simulink model "ACC_bicycleModel"  (R2022a)
settings: Solver=FixedStepAuto  StartTime=0.0  StopTime=T  RelTol=1e-3
values from neighbouring files (symbols this model uses):
  o0_ego_1 = 0    [PreRun.m]
  o0_lead = 0    [PreRun.m]
  t_gap = 1.4    [PreRun.m]
  Ts = 1e-2    (= 0.01)    [PreRun.m]
  v0_ego_1 = 20/9    (= 2.22222222222)    [PreRun.m]
  v0_lead = 25/9    (= 2.77777777778)    [PreRun.m]
  v_set = 30    [PreRun.m]
  x0_ego_1 = x0_lead - (10 + t_gap*v0_ego_1)    (= 56.8888888889)    [PreRun.m]
  x0_ego_2 = x0_ego_1 - (10 + t_gap*v0_ego_2)    (= 43.7777777778)    [PreRun.m]
  x0_lead = 70    [PreRun.m]
  y0_ego_1 = 0    [PreRun.m]
  y0_lead = 0    [PreRun.m]
libraries: robotmobilelib x3, mpcadaslib x2
settings Model: Creator=The MathWorks, Inc.  LastModifiedBy=SAMEER TALWAR
settings SolverCC: AlgebraicLoopSolver=TrustRegion
settings DataIOCC: ReturnWorkspaceOutputs=off
settings DebuggingCC: UnconnectedInputMsg=warning  UnconnectedOutputMsg=warning  UnconnectedLineMsg=warning  SFMachineParentedDataDiag=warning  ArithmeticOperatorsInVariantConditions=warning
settings SFSimCC: SimUseLocalCustomCode=off  CustomCodeUndefinedFunction=UseInterfaceOnly
settings RTWCC: RTWUseLocalCustomCode=off
settings CodeAppCC: StateflowObjectComments=on

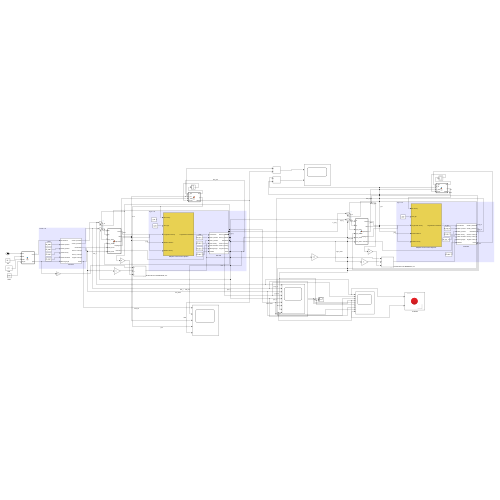
[thumbnail: Simulink's stored preview of the top-level diagram]
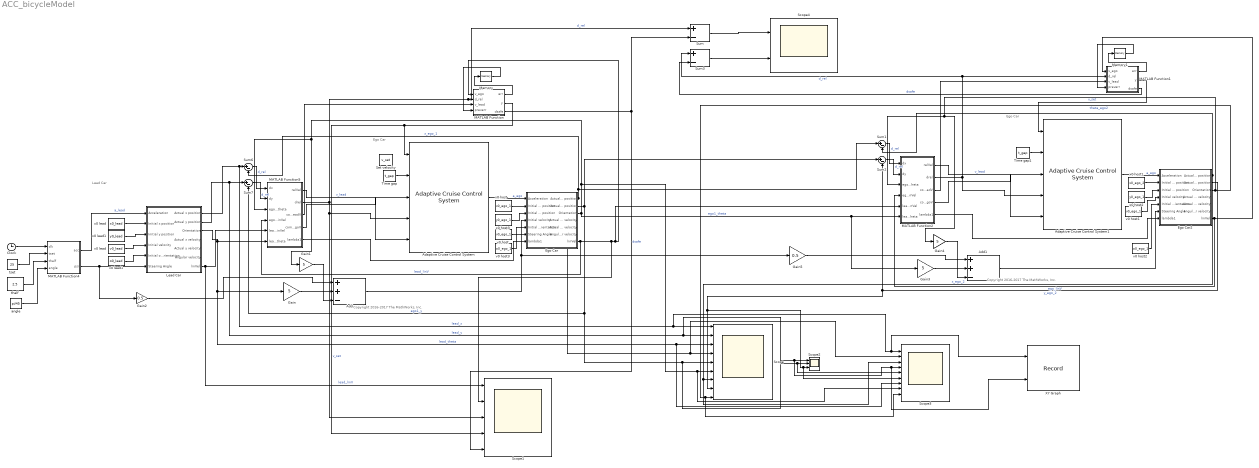
== system ACC_bicycleModel ==
  note: Lead Car
  note: Ego Car
  note: Copyright 2016-2017 The MathWorks, Inc.
  note: Ego Car
  note: Copyright 2016-2017 The MathWorks, Inc.
  Adaptive Cruise Control System : mpcadaslib/Adaptive Cruise Control System  EgoModel=tf(1,[0.5,1,0])  InitialEgoVelocity=20  DefaultSpacing=10  MaxVelocity=100  MinAcceleration=-30  amin_ext=off  MaxAcceleration=20  amax_ext=off  Ts=Ts  PredictionHorizon=30  ControllerBehavior=1.0  suboptimal=off  maxiter=10  datatypeopt=double  optmode=off  trackmode=off
  Adaptive Cruise Control System1 : mpcadaslib/Adaptive Cruise Control System  EgoModel=tf(1,[0.5,1,0])  InitialEgoVelocity=20  DefaultSpacing=10  MaxVelocity=100  MinAcceleration=-30  amin_ext=off  MaxAcceleration=20  amax_ext=off  Ts=Ts  PredictionHorizon=30  ControllerBehavior=1.0  suboptimal=off  maxiter=10  datatypeopt=double  optmode=off  trackmode=off
  Add : Sum  Inputs=++-
  Add1 : Sum  Inputs=++-
  Clock : Clock
  Ego Car : Subsystem
  Ego Car2 : Subsystem
  Gain{,1,3..4} (4 alike) : Gain  Gain=5
  Gain2 : Gain  Gain=0.5
  Gain5 : Gain  Gain=0.5
  Lead Car : Subsystem
  MATLAB Function : MATLAB Function  TreatAsAtomicUnit=on
  MATLAB Function1 : MATLAB Function  TreatAsAtomicUnit=on
  MATLAB Function2 : MATLAB Function  TreatAsAtomicUnit=on
  MATLAB Function4 : MATLAB Function  TreatAsAtomicUnit=on
  MATLAB Function5 : MATLAB Function  TreatAsAtomicUnit=on
  Memory : Memory
  Memory1 : Memory
  Scope : Scope  NumInputPorts=9
  Scope1 : Scope  NumInputPorts=5
  Scope2 : Scope  NumInputPorts=3
  Scope3 : Scope  NumInputPorts=9
  Scope4 : Scope  NumInputPorts=2
  Set velocity : Constant  Value=v_set  SampleTime=Ts
  Sum : Sum  Inputs=+-
  Sum{1..2,6..7} (4 alike) : Sum  Inputs=|+-
  Sum3 : Sum  Inputs=+-
  Time gap : Constant  Value=t_gap  SampleTime=Ts
  Time gap1 : Constant  Value=t_gap  SampleTime=Ts
  XY Graph : Record  FileSettingsInternal="{\"entries\":[{\"content\":{\"excelSettings\":{\"content\":{},\"type\":\"Streamout.ExcelSettings\"}},\"type\":\"Streamout.FileSettingStorage\",\"uuid\":\"e1ca2645-03e2-4b36-ae2b-66a36fe1bab2\"}],\"packageUris\":[\"http://schema.mathworks.com/mf0/streamout_blocks/R2020a\"],\"version\":\"1.0\"}"  Layout=[1 1]  SignalsInternal="{\"entries\":[{\"content\":{\"signals\":[{\"content\":{\"blockPath\":[\"ACC_bicycleModel/XY Graph\"],\"channel\":[],\"dimensions\":[1],\"domain\":\"ACC_bicycleModel/XY Graph\",\"lineColor\":\"#a2142f\",\"plots\":[1],\"port\":1,\"sid\":[],\"signalID\":18,\"signalName\":\"lead_x\"},\"type\":\"RecordBlkView.Signal\",\"uuid\":\"ab4e1985-af17-4664-8952-9c7faca9cf0c\"},{\"content\":{\"blockPath\":[\"ACC_bicycleModel/XY Graph\"],\"channel\":[],\"dimensions\":[1],\"domain\":\"ACC_bicycleModel/XY Graph\",\"lineColor\":\"#139fff\",\"plots\":[1],\"port\":2,\"sid\":[],\"signalID\":21,\"signalName\":\"lead_y\"},\"type\":\"RecordBlkView.Signal\",\"uuid\":\"8268d064-4b91-4bd3-a13e-a9de1dfc659a\"}]},\"type\":\"RecordBlkView.InputSignals\",\"uuid\":\"82ea261d-5a9d-4d47-9c53-a0f0462a1ab9\"}],\"packageUris\":[\"http://schema.mathworks.com/mf0/streamout_blocks/R2020a\"],\"version\":\"1.0\"}"  VisualizationBindings="{\"xyplotplugin\":{\"info\":[{\"series\":[{\"bindingParametersList\":[{\"parameter\":\"X-Axis\",\"signalID\":18,\"signalName\":\"lead_x\"},{\"parameter\":\"Y-Axis\",\"signalID\":21,\"signalName\":\"lead_y\"}],\"seriesID\":63900}],\"subplotID\":1}]}}"  CompatibilityTag=XY
  angle : Constant  Value=pi/45
  thalf : Constant  Value=2.5
  tset : Constant  Value=25
  v0 host : Constant  Value=v0_ego_1  SampleTime=Ts
  v0 host1 : Constant  Value=v0_ego_1  SampleTime=Ts
  v0 host2 : Constant  Value=o0_ego_1  SampleTime=Ts
  v0 host3 : Constant  Value=o0_ego_1  SampleTime=Ts
  v0 lead : Constant  Value=v0_lead  SampleTime=Ts
  v0 lead1 : Constant  Value=o0_lead  SampleTime=Ts
  x0 host : Constant  Value=x0_ego_1  SampleTime=Ts
  x0 host1 : Constant  Value=x0_ego_2  SampleTime=Ts
  x0 host2 : Constant  Value=y0_ego_1  SampleTime=Ts
  x0 host3 : Constant  Value=y0_ego_1  SampleTime=Ts
  x0 lead : Constant  Value=x0_lead  SampleTime=Ts
  x0 lead1 : Constant  Value=y0_lead  SampleTime=Ts
  wires:
  x0 lead/1 -> Lead Car/2(Initial x position)
  v0 lead/1 -> Lead Car/4(Initial velocity)
  x0 host/1 -> Ego Car/2(Initial x position)
  Adaptive Cruise Control System/1 -> Ego Car/1(Acceleration)  "a_ego"
  MATLAB Function5/2(drel) -> Sum/1, MATLAB Function/2(d_rel), Scope1/3, Adaptive Cruise Control System/4  "d_rel"
  Time gap/1 -> Adaptive Cruise Control System/2
  Ego Car/1(Actual x position) -> Sum1/1, Sum6/2, Scope3/2, Scope/4  "x_ego_1"
  MATLAB Function/2(y) -> Scope1/4, Adaptive Cruise Control System/1  "v_set"
  MATLAB Function4/1(acc) -> Lead Car/1(Acceleration)  "a_lead"
  MATLAB Function/1(err) -> Memory/1
  Memory/1 -> MATLAB Function/4(preverr)
  x0 host3/1 -> Ego Car/3(Initial y position)
  v0 host3/1 -> Ego Car/5(Initial orientation)
  Add/1 -> Gain5/1, Ego Car/6(Steering Angle)
  Clock/1 -> MATLAB Function4/1(clk)
  tset/1 -> MATLAB Function4/2(tset)
  thalf/1 -> MATLAB Function4/3(thalf)
  angle/1 -> MATLAB Function4/4(angle)
  MATLAB Function4/2(psi) -> Gain2/1, Lead Car/6(Steering Angle)
  x0 lead1/1 -> Lead Car/3(Initial y position)
  v0 lead1/1 -> Lead Car/5(Initial orientation)
  Lead Car/1(Actual x position) -> XY Graph/1, Scope3/1, Scope/1, Sum6/1  "lead_x"
  Lead Car/2(Actual y position) -> Scope3/4, XY Graph/2, Scope2/1, Scope/2, Sum7/1  "lead_y"
  Sum6/1 -> MATLAB Function5/1(dx)  "d_rel"
  Sum7/1 -> MATLAB Function5/2(dy)  "d_rel"
  Lead Car/7(linVel) -> MATLAB Function5/5(lead_linVel), Scope1/1  "lead_linV"
  Lead Car/3(Orientation) -> Scope3/7, Scope/3, Gain/1, MATLAB Function5/6(lead_theta)  "lead_theta"
  MATLAB Function5/1(relVel) -> Adaptive Cruise Control System/5  "v_lead"
  MATLAB Function5/3(compLeadV) -> MATLAB Function/3(v_lead)
  MATLAB Function5/4(compEgoV) -> Adaptive Cruise Control System/3
  MATLAB Function5/5(lambda1) -> Ego Car/7(lambda1)
  Gain/1 -> Add/2
  Gain1/1 -> Add/3
  Gain2/1 -> Add/1
  MATLAB Function/3(dsafe) -> Sum/2, Scope1/5  "dsafe"
  Ego Car/7(linVel) -> Scope1/2, MATLAB Function2/5(lead_linVel), MATLAB Function/1(v_ego), MATLAB Function5/4(ego_linVel)  "lead_linV"
  Ego Car2/2(Actual y position) -> Scope3/6, Scope2/3, Scope/8, Sum2/2  "y_ego_2"
  MATLAB Function2/5(lambda1) -> Ego Car2/7(lambda1)
  Gain3/1 -> Add1/2
  Gain4/1 -> Add1/3
  x0 host1/1 -> Ego Car2/2(Initial x position)
  Sum1/1 -> MATLAB Function2/1(dx)  "d_rel"
  Sum2/1 -> MATLAB Function2/2(dy)  "d_rel"
  MATLAB Function2/3(compLeadV) -> MATLAB Function1/3(v_lead)
  Ego Car2/3(Orientation) -> Scope3/9, Scope/9, Gain4/1, MATLAB Function2/3(ego_theta)  "theta_ego2"
  MATLAB Function1/2(y) -> Adaptive Cruise Control System1/1  "v_set"
  Ego Car/3(Orientation) -> Gain3/1, MATLAB Function2/6(lead_theta), Scope3/8, Scope/6, Gain1/1, MATLAB Function5/3(ego_theta)  "ego1_theta"
  v0 host2/1 -> Ego Car2/5(Initial orientation)
  x0 host2/1 -> Ego Car2/3(Initial y position)
  v0 host/1 -> Ego Car/4(Initial velocity)
  Ego Car/2(Actual y position) -> Sum2/1, Scope3/5, Scope2/2, Scope/5, Sum7/2  "ego1_y"
  MATLAB Function2/4(compEgoV) -> Adaptive Cruise Control System1/3
  Memory1/1 -> MATLAB Function1/4(preverr)
  MATLAB Function1/1(err) -> Memory1/1
  MATLAB Function2/1(relVel) -> Adaptive Cruise Control System1/5  "v_lead"
  Add1/1 -> Ego Car2/6(Steering Angle)
  Ego Car2/7(linVel) -> MATLAB Function1/1(v_ego), MATLAB Function2/4(ego_linVel)  "ego_linV"
  v0 host1/1 -> Ego Car2/4(Initial velocity)
  MATLAB Function2/2(drel) -> Adaptive Cruise Control System1/4, MATLAB Function1/2(d_rel), Sum3/1  "d_rel"
  Adaptive Cruise Control System1/1 -> Ego Car2/1(Acceleration)  "a_ego"
  Ego Car2/1(Actual x position) -> Sum1/2, Scope3/3, Scope/7  "x_ego_2"
  Time gap1/1 -> Adaptive Cruise Control System1/2
  Gain5/1 -> Add1/1
  Sum/1 -> Scope4/1
  MATLAB Function1/3(dsafe) -> Sum3/2  "dsafe"
  Sum3/1 -> Scope4/2

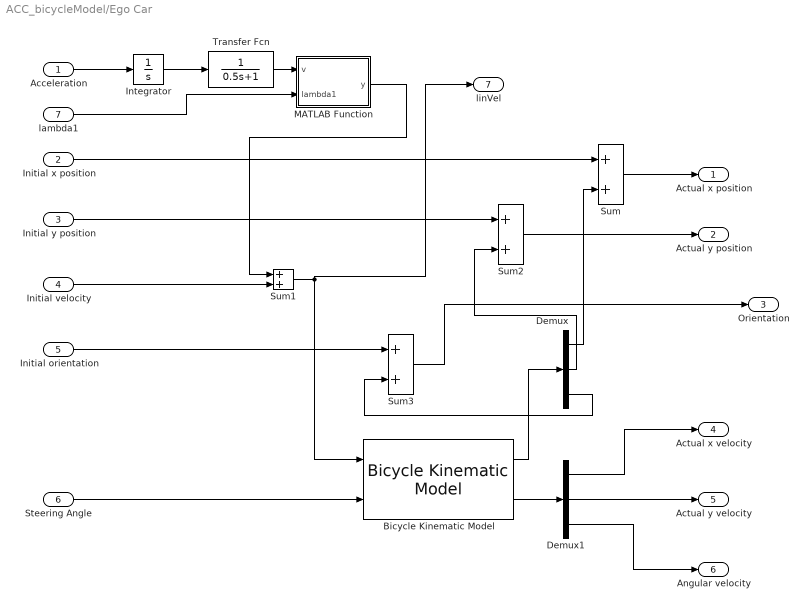
== system ACC_bicycleModel/Ego Car ==
  Acceleration : Inport
  Initial x position : Inport  Port=2
  Initial y position : Inport  Port=3
  Initial velocity : Inport  Port=4
  Initial orientation : Inport  Port=5
  Steering Angle : Inport  Port=6
  lambda1 : Inport  Port=7
  Bicycle Kinematic Model : robotmobilelib/Bicycle Kinematic Model  VehicleInputs=Vehicle Speed & Steering Angle  WheelBase=1  VehicleSpeedRange=[-inf inf]  MaxSteeringAngle=pi/4  InitialState=[0; 0; 0]  SimulateUsing=Interpreted execution
      settings: SourceProductBaseCode=RO
  Demux : Demux  Outputs=3
  Demux1 : Demux  Outputs=3
  Integrator : Integrator
  MATLAB Function : MATLAB Function  TreatAsAtomicUnit=on
  Sum{,1..3} (4 alike) : Sum
  Transfer Fcn : TransferFcn  Denominator=[0.5 1]
  Actual x position : Outport  VectorParamsAs1DForOutWhenUnconnected=off
  Actual y position : Outport  Port=2
  Orientation : Outport  Port=3
  Actual x velocity : Outport  Port=4  VectorParamsAs1DForOutWhenUnconnected=off
  Actual y velocity : Outport  Port=5
  Angular velocity : Outport  Port=6
  linVel : Outport  Port=7
  wires:
  Initial velocity/1 -> Sum1/2
  Sum/1 -> Actual x position/1
  Integrator/1 -> Transfer Fcn/1
  Acceleration/1 -> Integrator/1
  Initial x position/1 -> Sum/1
  Demux/1 -> Sum/2
  Bicycle Kinematic Model/1 -> Demux/1
  Sum1/1 -> linVel/1, Bicycle Kinematic Model/1
  Steering Angle/1 -> Bicycle Kinematic Model/2
  Bicycle Kinematic Model/2 -> Demux1/1
  Demux1/1 -> Actual x velocity/1
  Demux1/2 -> Actual y velocity/1
  Demux1/3 -> Angular velocity/1
  Initial y position/1 -> Sum2/1
  Demux/2 -> Sum2/2
  Sum2/1 -> Actual y position/1
  Initial orientation/1 -> Sum3/1
  Demux/3 -> Sum3/2
  Sum3/1 -> Orientation/1
  Transfer Fcn/1 -> MATLAB Function/1(v)
  lambda1/1 -> MATLAB Function/2(lambda1)
  MATLAB Function/1(y) -> Sum1/1

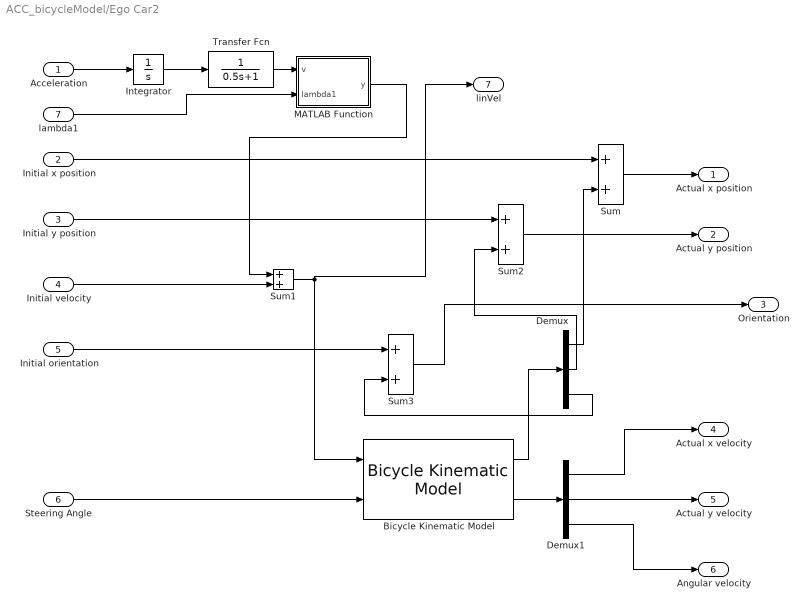
== system ACC_bicycleModel/Ego Car2 ==
  Acceleration : Inport
  Initial x position : Inport  Port=2
  Initial y position : Inport  Port=3
  Initial velocity : Inport  Port=4
  Initial orientation : Inport  Port=5
  Steering Angle : Inport  Port=6
  lambda1 : Inport  Port=7
  Bicycle Kinematic Model : robotmobilelib/Bicycle Kinematic Model  VehicleInputs=Vehicle Speed & Steering Angle  WheelBase=1  VehicleSpeedRange=[-inf inf]  MaxSteeringAngle=pi/4  InitialState=[0; 0; 0]  SimulateUsing=Interpreted execution
      settings: SourceProductBaseCode=RO
  Demux : Demux  Outputs=3
  Demux1 : Demux  Outputs=3
  Integrator : Integrator
  MATLAB Function : MATLAB Function  TreatAsAtomicUnit=on
  Sum{,1..3} (4 alike) : Sum
  Transfer Fcn : TransferFcn  Denominator=[0.5 1]
  Actual x position : Outport  VectorParamsAs1DForOutWhenUnconnected=off
  Actual y position : Outport  Port=2
  Orientation : Outport  Port=3
  Actual x velocity : Outport  Port=4  VectorParamsAs1DForOutWhenUnconnected=off
  Actual y velocity : Outport  Port=5
  Angular velocity : Outport  Port=6
  linVel : Outport  Port=7
  wires:
  Initial velocity/1 -> Sum1/2
  Sum/1 -> Actual x position/1
  Integrator/1 -> Transfer Fcn/1
  Acceleration/1 -> Integrator/1
  Initial x position/1 -> Sum/1
  Demux/1 -> Sum/2
  Bicycle Kinematic Model/1 -> Demux/1
  Sum1/1 -> linVel/1, Bicycle Kinematic Model/1
  Steering Angle/1 -> Bicycle Kinematic Model/2
  Bicycle Kinematic Model/2 -> Demux1/1
  Demux1/1 -> Actual x velocity/1
  Demux1/2 -> Actual y velocity/1
  Demux1/3 -> Angular velocity/1
  Initial y position/1 -> Sum2/1
  Demux/2 -> Sum2/2
  Sum2/1 -> Actual y position/1
  Initial orientation/1 -> Sum3/1
  Demux/3 -> Sum3/2
  Sum3/1 -> Orientation/1
  Transfer Fcn/1 -> MATLAB Function/1(v)
  lambda1/1 -> MATLAB Function/2(lambda1)
  MATLAB Function/1(y) -> Sum1/1

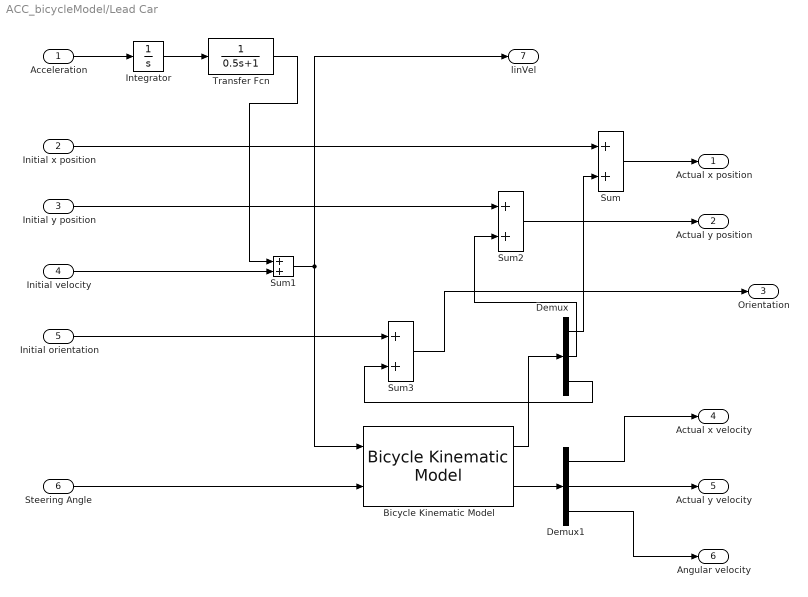
== system ACC_bicycleModel/Lead Car ==
  Acceleration : Inport
  Initial x position : Inport  Port=2
  Initial y position : Inport  Port=3
  Initial velocity : Inport  Port=4
  Initial orientation : Inport  Port=5
  Steering Angle : Inport  Port=6
  Bicycle Kinematic Model : robotmobilelib/Bicycle Kinematic Model  VehicleInputs=Vehicle Speed & Steering Angle  WheelBase=1  VehicleSpeedRange=[-inf inf]  MaxSteeringAngle=pi/4  InitialState=[0; 0; 0]  SimulateUsing=Interpreted execution
      settings: SourceProductBaseCode=RO
  Demux : Demux  Outputs=3
  Demux1 : Demux  Outputs=3
  Integrator : Integrator
  Sum{,1..3} (4 alike) : Sum
  Transfer Fcn : TransferFcn  Denominator=[0.5 1]
  Actual x position : Outport  VectorParamsAs1DForOutWhenUnconnected=off
  Actual y position : Outport  Port=2
  Orientation : Outport  Port=3
  Actual x velocity : Outport  Port=4  VectorParamsAs1DForOutWhenUnconnected=off
  Actual y velocity : Outport  Port=5
  Angular velocity : Outport  Port=6
  linVel : Outport  Port=7
  wires:
  Bicycle Kinematic Model/1 -> Demux/1
  Sum3/1 -> Orientation/1
  Steering Angle/1 -> Bicycle Kinematic Model/2
  Demux1/1 -> Actual x velocity/1
  Demux/1 -> Sum/2
  Demux/3 -> Sum3/2
  Demux1/2 -> Actual y velocity/1
  Initial orientation/1 -> Sum3/1
  Demux/2 -> Sum2/2
  Sum2/1 -> Actual y position/1
  Demux1/3 -> Angular velocity/1
  Bicycle Kinematic Model/2 -> Demux1/1
  Sum1/1 -> linVel/1, Bicycle Kinematic Model/1
  Integrator/1 -> Transfer Fcn/1
  Acceleration/1 -> Integrator/1
  Transfer Fcn/1 -> Sum1/1
  Initial y position/1 -> Sum2/1
  Sum/1 -> Actual x position/1
  Initial x position/1 -> Sum/1
  Initial velocity/1 -> Sum1/2

== matlab function ACC_bicycleModel/Ego Car/MATLAB Function ==
  data: y output; v input; lambda1 input
function y = fcn(v, lambda1)

y = v*sec(lambda1);

== matlab function ACC_bicycleModel/MATLAB Function ==
  data: err output; v_ego input; y output; d_rel input; v_lead input; preverr input; dsafe output
function [err,y,dsafe]= fcn(v_ego, d_rel, v_lead, preverr)
Kp = 5;
Kd = 20;
dsafe = 10 + (1.4*v_ego);
err = (d_rel - (10 + (1.4*v_ego)));
y = v_lead + Kp*err + Kd*(err-preverr);

== matlab function ACC_bicycleModel/Ego Car2/MATLAB Function ==
  data: y output; v input; lambda1 input
function y = fcn(v, lambda1)

y = v*sec(lambda1);

== matlab function ACC_bicycleModel/MATLAB Function1 ==
  data: err output; v_ego input; y output; d_rel input; v_lead input; preverr input; dsafe output
function [err,y,dsafe]= fcn(v_ego, d_rel, v_lead, preverr)
Kp = 5;
Kd = 20;
dsafe = 10 + (1.4*v_ego);
err = (d_rel - (10 + (1.4*v_ego)));
y = v_lead + Kp*err + Kd*(err-preverr);

== matlab function ACC_bicycleModel/MATLAB Function4 ==
  data: clk input; acc output; tset input; thalf input; angle input; psi output
function [acc,psi] = fcn(clk,tset,thalf, angle)
if clk>tset && clk<(tset+thalf)
    acc = angle;
elseif clk>(tset+thalf) && clk<(tset + 2*thalf)
    acc = 0;
else 
    acc = 0;
end
psi=0;

== matlab function ACC_bicycleModel/MATLAB Function5 ==
  data: relVel output; dx input; drel output; dy input; ego_theta input; ego_linVel input; lead_linVel input; lead_theta input; compLeadV output; compEgoV output; lambda1 output
function [relVel,drel,compLeadV, compEgoV, lambda1] = fcn(dx,dy, ego_theta, ego_linVel,lead_linVel, lead_theta)
drel = sqrt(dx^2 + dy^2);
lambda1 = atan(dy/dx) - ego_theta;
lambda2 = atan(dy/dx) - lead_theta;
relVel = lead_linVel*cos(lambda2) - ego_linVel*cos(lambda1);
compLeadV = lead_linVel*cos(lambda2);
compEgoV = ego_linVel*cos(lambda1);

== matlab function ACC_bicycleModel/MATLAB Function2 ==
  data: relVel output; dx input; drel output; dy input; ego_theta input; ego_linVel input; lead_linVel input; lead_theta input; compLeadV output; compEgoV output; lambda1 output
function [relVel,drel,compLeadV, compEgoV, lambda1] = fcn(dx,dy, ego_theta, ego_linVel,lead_linVel, lead_theta)
drel = sqrt(dx^2 + dy^2);
lambda1 = atan(dy/dx) - ego_theta;
lambda2 = atan(dy/dx) - lead_theta;
relVel = lead_linVel*cos(lambda2) - ego_linVel*cos(lambda1);
compLeadV = lead_linVel*cos(lambda2);
compEgoV = ego_linVel*cos(lambda1);
